simulink model "Second_order"  (R2021b)
settings: Solver=VariableStepAuto  StartTime=0.0  StopTime=20  RelTol=1e-3
undefined symbols (not defined in the file): Ts, U, Vmax
settings Model: Creator=11035  LastModifiedBy=11035

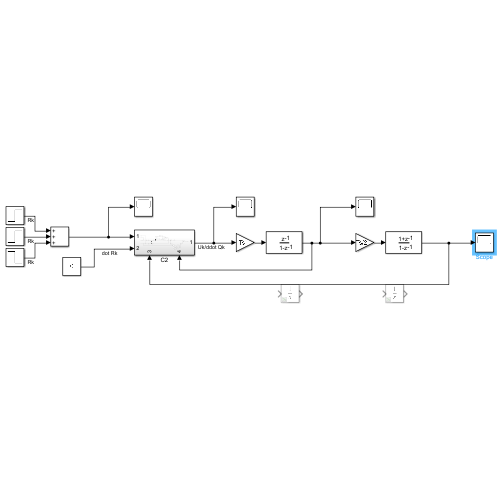
[thumbnail: Simulink's stored preview of the top-level diagram]
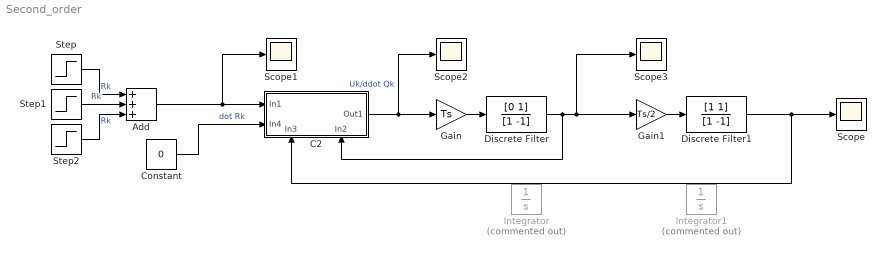
== system Second_order ==
  Add : Sum  Inputs=+++
  C2 : Subsystem
      settings: PortSchema="{\"entries\":[{\"content\":{\"sides\":[{\"content\":{\"connectorIds\":[\"In1\",\"In2\"]},\"type\":\"ConnectorPlacement.EquallySpacedRectSide\",\"uuid\":\"716dbc1c-49b2-4cb8-9978-582acac14571\"},{\"content\":{\"connectorIds\":[\"Out1\"],\"side\":\"RIGHT\"},\"type\":\"ConnectorPlacement.EquallySpacedRectSide\",\"uuid\":\"02ab29e9-5fcc-4cd5-9c74-177b5082cb9c\"},{\"content\":{\"connectorIds\":[],\"side\":\"TOP\"},\"type\":\"ConnectorPlacement.EquallySpacedRectSide\",\"uuid\":\"01e65ab7-ae67-4bc4-815c-31b93fbda65a\"},{\"content\":{\"connectorIds\":[\"In3\",\"In4\"],\"side\":\"BOTTOM\"},\"type\":\"ConnectorPlacement.EquallySpacedRectSide\",\"uuid\":\"7a24d1a6-7a93-4ed1-ab59-9b35f53416c1\"}]},\"type\":\"ConnectorPlacement.EquallySpacedConnector\",\"uuid\":\"504bdbd8-79dc-4418-b775-c54dc6ccf1a1\"}],\"packageUris\":[\"http://schema.mathworks.com/mf0/Connector/R2020b\"],\"version\":\"1.0\"}"
  Constant : Constant  Value=0
  Discrete Filter : DiscreteFilter  Numerator=[0 1]  Denominator=[1 -1]
  Discrete Filter1 : DiscreteFilter  Numerator=[1 1]  Denominator=[1 -1]
  Gain : Gain  Gain=Ts
  Gain1 : Gain  Gain=Ts/2
  Integrator : Integrator  Commented=on
  Integrator1 : Integrator  Commented=on
  Scope{,1..3} (4 alike) : Scope
  Step : Step  After=4  SampleTime=0.001
  Step1 : Step  Time=7  After=6  SampleTime=0.001
  Step2 : Step  Time=13  After=-12  SampleTime=0.001
  wires:
  C2/1(Out1) -> Gain/1, Scope2/1  "Uk/ddot Qk"
  Gain/1 -> Discrete Filter/1
  Constant/1 -> C2/2(In4)  "dot Rk"
  Discrete Filter/1 -> C2/4(In2), Gain1/1, Scope3/1
  Gain1/1 -> Discrete Filter1/1
  Discrete Filter1/1 -> C2/3(In3), Scope/1
  Step2/1 -> Add/3  "Rk"
  Step/1 -> Add/1  "Rk"
  Step1/1 -> Add/2  "Rk"
  Add/1 -> Scope1/1, C2/1(In1)

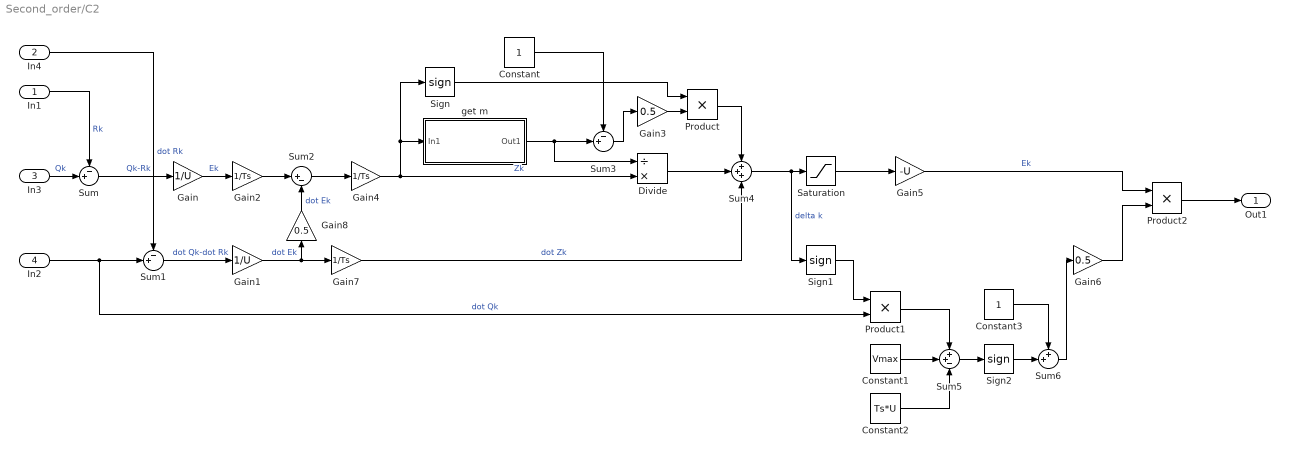
== system Second_order/C2 ==
  In1 : Inport
  In4 : Inport  Port=2
  In3 : Inport  Port=3
  In2 : Inport  Port=4
  Constant : Constant
  Constant1 : Constant  Value=Vmax
  Constant2 : Constant  Value=Ts*U
  Constant3 : Constant
  Divide : Product  Inputs=/*
  Gain : Gain  Gain=1/U
  Gain1 : Gain  Gain=1/U
  Gain2 : Gain  Gain=1/Ts
  Gain3 : Gain  Gain=0.5
  Gain4 : Gain  Gain=1/Ts
  Gain5 : Gain  Gain=-U
  Gain6 : Gain  Gain=0.5
  Gain7 : Gain  Gain=1/Ts
  Gain8 : Gain  Gain=0.5
  Product : Product
  Product1 : Product
  Product2 : Product
  Saturation : Saturate  UpperLimit=1  LowerLimit=-1
  Sign : Signum
  Sign1 : Signum
  Sign2 : Signum
  Sum : Sum  Inputs=-+|
  Sum1 : Sum  Inputs=-+|
  Sum2 : Sum  Inputs=|+-
  Sum3 : Sum  Inputs=-+|
  Sum4 : Sum  Inputs=+++
  Sum5 : Sum  Inputs=++-
  Sum6 : Sum  Inputs=++|
  get m : Subsystem
  Out1 : Outport
  wires:
  In1/1 -> Sum/1  "Rk"
  In3/1 -> Sum/2  "Qk"
  Sum/1 -> Gain/1  "Qk-Rk"
  Gain/1 -> Gain2/1  "Ek"
  In2/1 -> Product1/2, Sum1/2  "dot Qk"
  Sum1/1 -> Gain1/1  "dot Qk-dot Rk"
  Gain2/1 -> Sum2/1
  Sum2/1 -> Gain4/1
  Gain1/1 -> Gain7/1, Gain8/1  "dot Ek"
  Gain4/1 -> Sign/1, get m/1(In1), Divide/2  "Zk"
  Constant/1 -> Sum3/1
  Sum3/1 -> Gain3/1
  Gain3/1 -> Product/2
  Sign/1 -> Product/1
  Product/1 -> Sum4/1
  Divide/1 -> Sum4/2
  Sum4/1 -> Saturation/1, Sign1/1  "delta k"
  Sign1/1 -> Product1/1
  Constant1/1 -> Sum5/2
  Product1/1 -> Sum5/1
  Constant2/1 -> Sum5/3
  Sum5/1 -> Sign2/1
  Constant3/1 -> Sum6/1
  Sign2/1 -> Sum6/2
  Sum6/1 -> Gain6/1
  Saturation/1 -> Gain5/1
  Gain6/1 -> Product2/2
  Product2/1 -> Out1/1
  In4/1 -> Sum1/1  "dot Rk"
  Gain7/1 -> Sum4/3  "dot Zk"
  Gain5/1 -> Product2/1  "Ek"
  Gain8/1 -> Sum2/2  "dot Ek"
  get m/1(Out1) -> Divide/1, Sum3/2

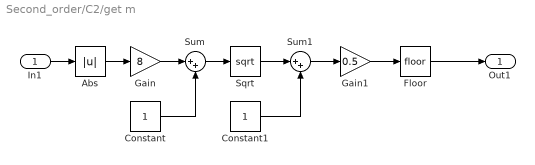
== system Second_order/C2/get m ==
  In1 : Inport
  Abs : Abs
  Constant : Constant
  Constant1 : Constant
  Floor : Rounding
  Gain : Gain  Gain=8
  Gain1 : Gain  Gain=0.5
  Sqrt : Sqrt  OutputSignalType=real  SaturateOnIntegerOverflow=on
  Sum : Sum  Inputs=|++
  Sum1 : Sum  Inputs=|++
  Out1 : Outport
  wires:
  In1/1 -> Abs/1
  Abs/1 -> Gain/1
  Gain/1 -> Sum/1
  Constant/1 -> Sum/2
  Gain1/1 -> Floor/1
  Floor/1 -> Out1/1
  Sum/1 -> Sqrt/1
  Sqrt/1 -> Sum1/1
  Sum1/1 -> Gain1/1
  Constant1/1 -> Sum1/2
